simulink model "Sim_Forcing_003h_expe_infra2"  (Simulink 7.4)
settings: Solver=FixedStepDiscrete  StartTime=0.0  StopTime=inf  FixedStep=0.004  RelTol=1e-3
undefined symbols (not defined in the file or in its folder): DiscIntNeverNeededParam
libraries: simulink x42, gt_rt_lib x30, xpcutilitieslib x9, xpclib x2, dspswit3 x1
(part 4 of 5)

== system Sim_Forcing_003h_expe_infra2/Joint Controller (May 7, 2015)/Inverse Kinematics June 22,2016 compatible_minirobot/Simplified Inverse Kinematics/Simplified Inverse Kin ==
  Vec : Inport  OutDataType=fixdt(1, 16)  OutScaling=2^0
  Enable : EnablePort
  Embedded MATLAB Function1 : Stateflow chart
  Out : Outport
  wires:
  Vec/1 -> Embedded MATLAB Function1/1(vec)
  Embedded MATLAB Function1/1(out) -> Out/1

== system Sim_Forcing_003h_expe_infra2/Joint Controller (May 7, 2015)/Inverse Kinematics May 6, 2015/Inverse Kinematics/full inverse kin ==
  vec : Inport
  Enable : EnablePort
  Embedded MATLAB Function : Stateflow chart
  out : Outport  OutDataType=fixdt(1, 16)  OutScaling=2^0
  wires:
  vec/1 -> Embedded MATLAB Function/1(vec)
  Embedded MATLAB Function/1(out) -> out/1

== system Sim_Forcing_003h_expe_infra2/Joint Controller (May 7, 2015)/Inverse Kinematics May 6, 2015/Simplified Inverse Kinematics/A1-A6 COM ==
  vec : Inport
  Demux1 : Demux  Outputs=7
  Ground : Ground
  Ground1 : Ground
  Ground2 : Ground
  Mux1 : Mux  Inputs=6
  Terminator{,1..3} (4 alike) : Terminator
  A1-A6 COM : Outport
  wires:
  Demux1/2 -> Mux1/2
  Demux1/3 -> Mux1/3
  Demux1/5 -> Mux1/5
  Ground/1 -> Mux1/1
  Ground1/1 -> Mux1/4
  Ground2/1 -> Mux1/6
  Demux1/1 -> Terminator/1
  Demux1/4 -> Terminator1/1
  Demux1/6 -> Terminator2/1
  Demux1/7 -> Terminator3/1
  Mux1/1 -> A1-A6 COM/1
  vec/1 -> Demux1/1

== system Sim_Forcing_003h_expe_infra2/Joint Controller (May 7, 2015)/Inverse Kinematics May 6, 2015/Simplified Inverse Kinematics/Simplified Inverse Kin ==
  Vec : Inport  OutDataType=fixdt(1, 16)  OutScaling=2^0
  Enable : EnablePort
  Embedded MATLAB Function1 : Stateflow chart
  Out : Outport
  wires:
  Vec/1 -> Embedded MATLAB Function1/1(vec)
  Embedded MATLAB Function1/1(out) -> Out/1

== matlab function Breaking_Control 20/07/15/Move UP1/add x_offset/Embedded MATLAB Function ==
  data: dx input double; set_out output double; set_in input double
function set_out = add_x_offset(dx, set_in)
%#eml

set_out = set_in;
set_out(3,1) = set_in(3,1) + dx;

== matlab function Breaking_Control 20/07/15/Timeline/Embedded MATLAB Function ==
  data: u input double; y output double; flag_in input double; ac_in input double; ac_out output double
function [y,ac_out]  = fcn(u,flag_in,ac_in)
%#eml
ac_out=ac_in;

if(u>0.2)
    ac_out=1;
    y=1;
else
if(ac_out==1)
    y=1;
    ac_out=1;
else
    y=0;
    ac_out=0;
end    
end

if(flag_in==1)
    ac_out=0;
    y=0;    
end



end

== matlab function Breaking_Control 20/07/15/Embedded MATLAB Function2 ==
  data: com_or input double; T output double size=1; threshold input double; flag_z output double
function [T,flag_z]  = check_angle(com_or,threshold)
%#eml
sum=com_or(1)+com_or(2)+com_or(3);

if(abs(sum)>threshold)
    T=10;
    flag_z=1;
else
    T=5;
    flag_z=0;
    
end

== matlab function Breaking_Control 20/07/15/Timeline/Embedded MATLAB Function2 ==
  data: stim_time input double; t_bool output uint8 size=1; flag_z input double
function t_bool   = adjust_time(stim_time,flag_z)
%#eml

if(flag_z)
    if(stim_time<50)
        t_bool=true;
    else
        t_bool=false;
    end
    
else
    if(stim_time<40)
        t_bool=true;
    else
        t_bool=false;
    end
  
end

== matlab function Joint Controller (May 7, 2015)/Forward Kinematics/Embedded MATLAB Function ==
  data: vec input double; out output uint8
function out = ForKinSim( vec )
%--------------------------------------------------------------------------
%
%   This function solves the FORWARD kinematics of the 6-DOF KUKA arm and
%   wrist. This is the  version,
%   embedded in Simulink. The input and output are vectors that include the
%   list of parameters as defined herafter
%
%       *** Input variables, vec(1:13) ***
%
%   vec(1: 3)    POS         Room coordinates of flange, NED in cm
%   vec(4: 6)    EUL_ANG     Euler angles of the flange, phi, theta, psi, in deg
%   vec(1:6)     J_ANG_0     The joint angles, in deg
%
%       *** Output Variables ***
%
%   out(1: 3)    POS         Room coordinates of flange, NED in cm
%   out(4: 6)    EUL_ANG     Euler angles of the flange, phi, theta, psi, in deg
%
%   The North_East_Down convention is used and psi, theta, phi rotation
%   sequence; A2, A3, A5 are up positive and A4, A6 right rotation positive
%   Note that this is different from the KUKA convention
%
%   Written by Arthur J. Grunwald, Nov. 23, 2014
%
%--------------------------------------------------------------------------
%#eml

DTR = pi/180.;
RTD = 180/pi;

% reload variables
% the algorithm works in rad, so ang is in rad
J_ANG       = vec(1:6);   % Initial guess of the joint angles, in deg
ang         = J_ANG*DTR;

% reserve place for output
out = zeros(6,1);

% define length of arms
l1          = 50.;   % arm length in cm
l2          = 130.;
l3          = 66.;
l4          = 36.5;
l5          = 29.;
d           = 5.5;             % vertical offset of the center line of
% joint 4 from centerline of arm A3
Height_A2   = 104.5 + 106;     % height link A2 above the ground


% 4x4 Transfer matrices, include both rotation and translation

ang = adjust_ang( ang ); % ang is brought in the range +-pi
A1 = ang(1);
A2 = ang(2);
A3 = ang(3);
A4 = ang(4);
A5 = ang(5);
A6 = ang(6);

CA1 = cos(A1);
SA1 = sin(A1);
CA2 = cos(A2);
SA2 = sin(A2);
CA3 = cos(A3);
SA3 = sin(A3);
CA4 = cos(A4);
SA4 = sin(A4);
CA5 = cos(A5);
SA5 = sin(A5);
CA6 = cos(A6);
SA6 = sin(A6);

D1 = [CA1 -SA1 0 0; SA1 CA1 0 0; 0 0 1 0;  0 0 0 1];
D2 = [CA2 0 SA2 l1; 0 1 0 0; -SA2 0 CA2 0; 0 0 0 1];
D3 = [CA3 0 SA3 l2; 0 1 0 0; -SA3 0 CA3 0; 0 0 0 1];
D4 = [1 0 0 l3; 0 CA4 -SA4 0; 0 SA4 CA4 d; 0 0 0 1];
D5 = [CA5 0 SA5 l4; 0 1 0 0; -SA5 0 CA5 0; 0 0 0 1];
D6 = [1 0 0 l5; 0 CA6 -SA6 0; 0 SA6 CA6 0; 0 0 0 1];

% cut out the 3x3 DCM's for each of the transfer matrices
% Note that the DCM is for rotation from b->e
E1 = D1(1:3,1:3);
E2 = D2(1:3,1:3);
E3 = D3(1:3,1:3);
E4 = D4(1:3,1:3);
E5 = D5(1:3,1:3);
E6 = D6(1:3,1:3);

% --- computed position from links A1-A6 ---

x_cabin = [0; 0; 0];    % x,y,z cabin reference point (cm)
% to which the translation is made
x6 = [x_cabin; 1];
p = D1*D2*D3*D4*D5*D6*x6;
pos = p(1:3);        % position of the cabin reference point in the
% NED system (cm)

% computed Euler angles from links A1-A6
% Euler matrices for rotation from e->b (note the transpose)
E = E6'*E5'*E4'*E3'*E2'*E1';
eul_ang = DCM2Eul( E );

% place into output vector
out(1:3,1) = pos-[0;0;Height_A2];
out(4:6,1) = RTD*eul_ang;

end

== matlab function Joint Controller (May 7, 2015)/Inverse Kinematics May 6, 2015/Inverse Kinematics/full inverse kin/Embedded MATLAB Function ==
  data: vec input double; out output double
function out = InvKinSim( vec )
%--------------------------------------------------------------------------
%
%   This function solves the inverse kinematics of the 6-DOF KUKA arm and
%   wrist by means of an iterative algorithm. This is the  version,
%   embedded in Simulink. The input and output are vectors that include the
%   list of parameters as defined herafter
%
%       *** Input variables, vec(1:13) ***
%
%   vec(1: 3)    POS         Room coordinates of flange, NED in cm
%   vec(4: 6)    EUL_ANG     Euler angles of the flange, phi, theta, psi, in deg
%   vec(7:12)    J_ANG_0     Initial guess of the joint angles, in deg
%
%       *** Output Variables ***
%
%   out(1:6)  J_ANG          The six joint angles after convergence
%   out(7)    N, error code  Number of iterations, when negative, it is an
%                            error code:
%                               -1 no convergence
%                               -2 out of reach of joints
%                               -3 joint angles exceeded
%
%   The North_East_Down convention is used and psi, theta, phi rotation
%   sequence; A2, A3, A5 are up positive and A4, A6 right rotation positive
%   Note that this is different from the KUKA convention
%
%   Written by Arthur J. Grunwald, Nov. 14, 2014
%   Re-written for Simulink embedded, Nov. 20, 2014
%
%--------------------------------------------------------------------------
%#eml
DTR = pi/180.;
RTD = 180/pi;

% reload variables
POS         = vec(1: 3);   % Room coordinates of flange, NED in cm
EUL_ANG     = vec(4: 6);   % Euler angles of the flange, phi, theta, psi, in deg
J_ANG_0     = vec(7:12);   % Initial guess of the joint angles, in deg
out         = zeros(7,1);  % reserve place for out

% soft limits on the links (NED convention)

% SL = [   175    130     88    200    61    200
%         -175    -20    -88   -200   -61   -200];

% Dec. 6, 2014: A2 and A3 limits changed to KUKA hardware
% May 7,2015 soft limits on the links (NED convention)
SL = [   159    129     87      349    60    349
        -159    -19    -87     -349   -60   -349];

% define length of arms
l1          = 50.;   % arm length in cm
l2          = 130.;
l3          = 66.;
l4          = 36.5;
l5          = 29.;
d           = 5.5;             % vertical offset of the center line of
% joint 4 from centerline of arm A3
Height_A2   = 104.5 + 106;     % height link A2 above the ground

% offset the height so that level zero is now at the height of the A2 joint
POS(3) = POS(3) + Height_A2;

% set initial guess; the algorithm works in rad, so ang is in rad
N = 0;
ang = J_ANG_0*DTR;

% check for maximum range of arm links and exit with n = 2 when exceeded
L = l2 + l3 + l4 + l5;
R = sqrt(L^2 - POS(3)^2) + l1;
R1 = sqrt(POS(1)^2 + POS(2)^2);
if R1 > R-5;
    out(1:6,1) = J_ANG_0; % return vector as is
    out(7,1)   = -2;
    return
end

%--------------------------------
% 	start of iterative loop
%--------------------------------

while(1)
    
    % 4x4 Transfer matrices, include both rotation and translation
    
    ang = adjust_ang( ang ); % ang is brought in the range +-pi
    A1 = ang(1);
    A2 = ang(2);
    A3 = ang(3);
    A4 = ang(4);
    A5 = ang(5);
    A6 = ang(6);
    
    CA1 = cos(A1);
    SA1 = sin(A1);
    CA2 = cos(A2);
    SA2 = sin(A2);
    CA3 = cos(A3);
    SA3 = sin(A3);
    CA4 = cos(A4);
    SA4 = sin(A4);
    CA5 = cos(A5);
    SA5 = sin(A5);
    CA6 = cos(A6);
    SA6 = sin(A6);
    
    D1 = [CA1 -SA1 0 0; SA1 CA1 0 0; 0 0 1 0;  0 0 0 1];
    D2 = [CA2 0 SA2 l1; 0 1 0 0; -SA2 0 CA2 0; 0 0 0 1];
    D3 = [CA3 0 SA3 l2; 0 1 0 0; -SA3 0 CA3 0; 0 0 0 1];
    D4 = [1 0 0 l3; 0 CA4 -SA4 0; 0 SA4 CA4 d; 0 0 0 1];
    D5 = [CA5 0 SA5 l4; 0 1 0 0; -SA5 0 CA5 0; 0 0 0 1];
    D6 = [1 0 0 l5; 0 CA6 -SA6 0; 0 SA6 CA6 0; 0 0 0 1];
    
    % cut out the 3x3 DCM's for each of the transfer matrices
    % Note that the DCM is for rotation from b->e
    E1 = D1(1:3,1:3);
    E2 = D2(1:3,1:3);
    E3 = D3(1:3,1:3);
    E4 = D4(1:3,1:3);
    E5 = D5(1:3,1:3);
    E6 = D6(1:3,1:3);
    
    % --- computed position from links A1-A6 ---
    
    %----------------------------------------------------------------------
    %   In order to move a point in the cabine in 6-DOF rather than the
    %   endplate, define the coordinates of that point in x_cabin
    %----------------------------------------------------------------------
    x_cabin = [0; 0; 0];    % x,y,z cabin reference point (cm)
    
    x6 = [x_cabin; 1];
    p = D1*D2*D3*D4*D5*D6*x6;
    pos = p(1:3);           % position of the cabin reference point in the
    % NED system (cm)
    
    % computed Euler angles from links A1-A6
    % Euler matrices for rotation from e->b (note the transpose)
    E = E6'*E5'*E4'*E3'*E2'*E1';
    eul_ang = DCM2Eul( E );
    
    % determine the vectors of rotation of the endplate in e-system
    % for each one of the links; this is a 3x6 matrix, when multiplied
    % with the vector of the joint angles, it will give the vector
    % of rotation of the endplate (and also of the cabin reference point)
    % in the NED system
    
    e6 = E1*E2*E3*E4*E5*[1 0 0]'; % x-axis
    e5 = E1*E2*E3*E4*   [0 1 0]'; % y-axis
    e4 = E1*E2*E3*      [1 0 0]'; % x-axis
    e3 = E1*E2*         [0 1 0]'; % y-axis
    e2 = E1*            [0 1 0]'; % y-axis
    e1 = eye(3)*        [0 0 1]'; % z-axis
    
    e = [e1 e2 e3 e4 e5 e6];
    
    % in order to see the changes in phi, theta, psi that this rotation
    % vector causes, we have to transform e->b first in yaw and after that
    % in pitch
    cs_psi = cos(eul_ang(3));
    sn_psi = sin(eul_ang(3));
    cs_tet = cos(eul_ang(2));
    sn_tet = sin(eul_ang(2));
    
    PSI = [cs_psi sn_psi 0; -sn_psi cs_psi 0; 0 0 1];
    TET = [cs_tet 0 -sn_tet; 0 1 0; sn_tet 0 cs_tet];
    e = TET*PSI*e;
    
    
    
    % the derivatives of D1-D6 for eah one of the link angles
    dD1 = [-SA1 -CA1 0 0; CA1 -SA1 0 0; 0 0 0 0; 0 0 0 0];
    dD2 = [-SA2 0 CA2 0; 0 0 0 0; -CA2 0 -SA2 0; 0 0 0 0];
    dD3 = [-SA3 0 CA3 0; 0 0 0 0; -CA3 0 -SA3 0; 0 0 0 0];
    dD4 = [0 0 0 0; 0 -SA4 -CA4 0; 0 CA4 -SA4 0; 0 0 0 0];
    dD5 = [-SA5 0 CA5 0; 0 0 0 0; -CA5 0 -SA5 0; 0 0 0 0];
    dD6 = [0 0 0 0; 0 -SA6 -CA6 0; 0 CA6 -SA6 0; 0 0 0 0];
    
    % Hessian Matrix H; the inverse of this matrix determines the link
    % angle speed as a function of the speed of x,y,z and the speed of the
    % Euler angles
    
    h1 = dD1*D2*D3*D4*D5*D6*x6;
    h2 = D1*dD2*D3*D4*D5*D6*x6;
    h3 = D1*D2*dD3*D4*D5*D6*x6;
    h4 = D1*D2*D3*dD4*D5*D6*x6;
    h5 = D1*D2*D3*D4*dD5*D6*x6;
    h6 = D1*D2*D3*D4*D5*dD6*x6;
    
    h = [h1 h2 h3 h4 h5 h6]; % this 3x6 is th upper half of H
    H = [h(1:3,:); e];       % the lower 3x6 half is the matrix e
    
    d_ang = inv(H) * [( POS - pos ); (DTR*EUL_ANG - eul_ang)];
    ang = ang + d_ang;
    ang = adjust_ang( ang );
    if(norm(d_ang) < 1.e-6)
        J_ANG = RTD*adjust_ang( ang );
        out(1:6,1) = J_ANG;
        out(7,1)   = N;
        break;
    end
    N = N + 1;
    
    % if more than 10 iterations, no convergence
    if N > 10
        out(1:6) = J_ANG_0; % return vector as is
        out(7)   = -1;
        return;
    end
end

% tests whether the links are within the set soft limits
for i = 1 : 6
    if J_ANG(i) >= SL(1,i)
        out(7,1) = -3;
        return;
    elseif J_ANG(i) <= SL(2,i)
        out(7,1) = -3;
        return;
    end
end

end

== matlab function Joint Controller (May 7, 2015)/Inverse Kinematics May 6, 2015/Simplified Inverse Kinematics/Simplified Inverse Kin/Embedded MATLAB Function1 ==
  data: vec input double; out output double
function out = SimpleInvKin( vec )

% We use the NED convention
% This algorithm has a closed form solution and is based on the cosine rule
% However, due to the offset of the centerline of link A4 55 mm below the
% center of rotation of link A3, some small corrections have to be made;
% this is done iteratively by means of a second-order scheme.
% The gist of this routine is to show tha identical results are obtained
% with the fully-fledged 6-DOF inverse algorithm.
%
% The algorithm is also used for computing an initial guess for the
% fully-fledged inverse kinematics algorithm
% The initial guess uses only links A1, A2, A3 and assumes that the
% cabin at the end is straight and level and aligned with the arm
% Thus A4 and A6 are zero and A5 is A2 + A3
%
%   out(7) includes the parameter N
%       N > 0           the number of iterations needed to converge
%       N = -1          the iterative algorithm does not converge
%       N = -2          out of reachable limits
%       N -10<N<-30     upper limit of one of the joints A1-A6 exceeded
%       N -100<N<-110   upper limit of one of the joints A1-A6 exceeded
%
%   Written by Arthur Grunwald, November 11, 2014
%   Added correction because of offset of link A4, Dec 2, 2014
%   Added theta degree-of-freedom April 14, 2015
%   Modified the iterative scheme to second order NR scheme April 24, 2015
%   Modified FAR and CLOSE checks with intersecting circles May 6, 2015

RTD = 180/pi;
DTR = pi/180;

% May 7,2015 soft limits on the links (NED convention)
SL = [   159    129     87      349    60    349
        -159    -19    -87     -349   -60   -349];

% define length of the links

l1          = 50.;   % arm length in cm
l2          = 130.;
l3          = 66.;
l4          = 36.5;
l5          = 29.;
offset      = 5.5;             % vertical offset of the center line of
% joint 4 from centerline of arm A3
% joint 4 from centerline of arm A3
Height_A2   = 104.5 + 106;     % height link A2 above the ground

x = vec(1);
y = vec(2);
z = vec(3);

theta = vec(5);
cos_theta = cos(DTR*vec(5));
sin_theta = sin(DTR*vec(5));

N = 1;
out = zeros(7,1);

% compute dimensions of triangle
l = sqrt(x*x + y*y);
e = l - l1 - l5*cos_theta;
h = -(Height_A2 + z)-l5*sin_theta;
d = sqrt(e^2 + h^2);

% check whether the FAR location of C is reachable
b = l2;
c = l3 + l4;
margin = 5; % margin is 5 cm
if d > b + c - margin
    out(1:6,1) = vec(7:12); % return angles 'as is'
    out(3,1) = -90;
    out(7,1) = -2;
    return
end

% check whether the CLOSE location of C is reachable
if d + c - margin < b
    out(1:6,1) = vec(7:12); % return angles 'as is'
    out(3,1) = -90;
    out(7,1) = -2;
    return
end

% This iterative loop serves to correct for the offset of link A4
% A first good guess is to assume that beta is initially 90 deg
% A second-order scheme is used

A3 = vec(9);
beta = A3 + 180.;

while(1)
    
    sin_beta = sin(beta*DTR);
    sin2_beta = sin_beta*sin_beta;
    cos_beta = cos(beta*DTR);
    
    b = l2 - offset/sin_beta;
    c = l3 + l4 - offset*cos_beta/sin_beta;
    
    db_dbeta = offset * cos_beta/sin2_beta;
    dc_dbeta = offset/sin2_beta;
    
    A = (b*b + c*c - d*d);
    B = (2*b*c);
    dA_dbeta = (2*b*db_dbeta + 2*c*dc_dbeta);
    dB_dbeta = 2*(db_dbeta*c + b*dc_dbeta);
    eps = cos_beta - A/B;
    deps_dbeta = -sin_beta - (dA_dbeta*B - A*dB_dbeta)/B^2;
    dbeta = -RTD*eps/deps_dbeta;
    beta = beta + dbeta;
    
    if abs(dbeta) < 1.e-5
        break
    end
    N = N + 1;
    if N > 100
        N = -2;
        out(1:6,1) = vec(7:12); % return angles 'as is'
        out(3,1) = -90;
        out(7,1) = N;
        break;
    end
end

% employ cosine rule on angles alpha and beta of triangle
cos_alpha = (b*b + d*d - c*c)/(2*b*d);

alpha = RTD*acos(cos_alpha);
delta = RTD*atan2(h, e);

% the link angles
A1 = RTD*atan2(y, x);
A2 = alpha + delta;
A3 = beta - 180;
A4 = 0;
A5 = -(A2 + A3) + theta;
A6 = 0;

J_ANG = [A1 A2 A3 A4 A5 A6]';
out(1:6,1) = J_ANG;

% tests whether the links are within the set soft limits
for i = 1 : 6
    if J_ANG(i) >= SL(1,i)
        N = -10-i;
    elseif J_ANG(i) <= SL(2,i)
        N = -100-i;
    end
end

out(7,1) = N;

end

== matlab function Breaking_Control 20/07/15/Move UP1/curve ==
  data: set input double; psi_set input double; x output double; fraction input double; z output double; psi output double; c output double; z_p output double
function [x, z, psi, c, z_p] = curve(set, psi_set, fraction)
%#eml
%**************************************************************************
%
% for fitting a parabolic curve through 3 points
%
%   set is a 3 x 2 matrix that include:
%       (x1, z1)
%       (x2, z2)
%       (x3, z3)
%
%   z is the abcis and x the ordinate of the curve
%   fraction runs from 0 to 1
%
%**************************************************************************

z_p = set(:,2);
x_p = set(:,1);

A = [z_p.*z_p z_p ones(3,1)];
c = A\x_p;

z = fraction*(z_p(3) - z_p(1)) + z_p(1);

x = [z.*z z 1]*c;

psi = fraction * psi_set;

== matlab function Joint Controller (May 7, 2015)/Inverse Kinematics June 22,2016 compatible_minirobot/Embedded MATLAB Function ==
  data: J_ANG_COURANTS input double; SCALED_J_ANG output double; J_ANG_ANCIENS input double
function SCALED_J_ANG  = LimitesCinematiqes(J_ANG_COURANTS, J_ANG_ANCIENS)
%#eml

A1C=J_ANG_COURANTS(1);      A1A=J_ANG_ANCIENS(1);
A2C=J_ANG_COURANTS(2);      A2A=J_ANG_ANCIENS(2);
A3C=J_ANG_COURANTS(3);      A3A=J_ANG_ANCIENS(3);
A4C=J_ANG_COURANTS(4);      A4A=J_ANG_ANCIENS(4);
A5C=J_ANG_COURANTS(5);      A5A=J_ANG_ANCIENS(5);
A6C=J_ANG_COURANTS(6);      A6A=J_ANG_ANCIENS(6);

BCtheta1=0.2734; BCtheta2=0.228; BCtheta3=0.276;
BCtheta45=0.304; BCtheta6=0.48;   
%---THETA1----------------------
delta1=A1C-A1A;
if(abs(delta1)> BCtheta1)
    Theta1=A1A+sign(delta1)*BCtheta1;
else
    Theta1=A1C;
end

%---THETA2----------------------
delta2=A2C-A2A;
if(abs(delta2)> BCtheta2)
    Theta2=A2A+sign(delta2)*BCtheta2;
else
    Theta2=A2C;
end
%---THETA3----------------------
delta3=A3C-A3A;
if(abs(delta3)> BCtheta3)
    Theta3=A3A+sign(delta3)*BCtheta3;
else
    Theta3=A3C;
end

%---THETA4----------------------
delta4=A4C-A4A;
if(abs(delta4)> BCtheta45)
    Theta4=A4A+sign(delta4)*BCtheta45;
else
    Theta4=A4C;
end
%---THETA5----------------------
delta5=A5C-A5A;
if(abs(delta5)> BCtheta45)
    Theta5=A5A+sign(delta5)*BCtheta45;
else
    Theta5=A5C;
end
%---THETA6----------------------
delta6=A6C-A6A;
if(abs(delta6)> BCtheta6)
    Theta6=A6A+sign(delta6)*BCtheta6;
else
    Theta6=A6C;
end
SCALED_J_ANG=[Theta1, Theta2, Theta3, Theta4, Theta5, Theta6];
end

== matlab function Breaking_Control 20/07/15/Timeline/Embedded MATLAB Function1 ==
  data: stim_time input double; t_bool output double size=1; flag_z input double
function t_bool   = adjust_time(stim_time,flag_z)
%#eml

if(flag_z)
    if(stim_time>=50)
        t_bool=true;
    else
        t_bool=false;
    end
    
else
    if(stim_time>=40)
        t_bool=true;
    else
        t_bool=false;
    end
  
end

== matlab function Breaking_Control 20/07/15/Timeline/Embedded MATLAB Function3 ==
  data: stim_time input double; t_bool output double size=1; flag_z input double
function t_bool   = adjust_time(stim_time,flag_z)
%#eml

if(flag_z)
    if(stim_time>=60)
        t_bool=true;
    else
        t_bool=false;
    end
    
else
    if(stim_time>=50)
        t_bool=true;
    else
        t_bool=false;
    end
  
end

== matlab function Breaking_Control 20/07/15/Timeline/Embedded MATLAB Function4 ==
  data: stim_time input double; t_bool output double size=1; flag_z input double
function t_bool   = adjust_time(stim_time,flag_z)
%#eml

if(flag_z)
    if(stim_time<30)
        t_bool=true;
    else
        t_bool=false;
    end
    
else
    if(stim_time<20)
        t_bool=true;
    else
        t_bool=false;
    end
  
end

== matlab function Joint Controller (May 7, 2015)/Inverse Kinematics June 22,2016 compatible_minirobot/Inverse Kinematics/full inverse kin/Embedded MATLAB Function ==
  data: vec input double; out output double
function out = InvKinSim( vec )
%--------------------------------------------------------------------------
%
%   This function solves the inverse kinematics of the 6-DOF KUKA arm and
%   wrist by means of an iterative algorithm. This is the  version,
%   embedded in Simulink. The input and output are vectors that include the
%   list of parameters as defined herafter
%
%       *** Input variables, vec(1:13) ***
%
%   vec(1: 3)    POS         Room coordinates of flange, NED in cm
%   vec(4: 6)    EUL_ANG     Euler angles of the flange, phi, theta, psi, in deg
%   vec(7:12)    J_ANG_0     Initial guess of the joint angles, in deg
%
%       *** Output Variables ***
%
%   out(1:6)  J_ANG          The six joint angles after convergence
%   out(7)    N, error code  Number of iterations, when negative, it is an
%                            error code:
%                               -1 no convergence
%                               -2 out of reach of joints
%                               -3 joint angles exceeded
%
%   The North_East_Down convention is used and psi, theta, phi rotation
%   sequence; A2, A3, A5 are up positive and A4, A6 right rotation positive
%   Note that this is different from the KUKA convention
%
%   Written by Arthur J. Grunwald, Nov. 14, 2014
%   Re-written for Simulink embedded, Nov. 20, 2014
%
%--------------------------------------------------------------------------
%#eml
DTR = pi/180.;
RTD = 180/pi;

% reload variables
POS         = vec(1: 3);   % Room coordinates of flange, NED in cm
EUL_ANG     = vec(4: 6);   % Euler angles of the flange, phi, theta, psi, in deg
J_ANG_0     = vec(7:12);   % Initial guess of the joint angles, in deg
out         = zeros(7,1);  % reserve place for out

% soft limits on the links (NED convention)

% SL = [   175    130     88    200    61    200
%         -175    -20    -88   -200   -61   -200];

% Dec. 6, 2014: A2 and A3 limits changed to KUKA hardware
% May 7,2015 soft limits on the links (NED convention)
SL = [   159    129     87      349    60    349
        -159    -19    -87     -349   -60   -349];

% define length of arms
l1          = 50.;   % arm length in cm
l2          = 130.;
l3          = 66.;
l4          = 36.5;
l5          = 29.;
d           = 5.5;             % vertical offset of the center line of
% joint 4 from centerline of arm A3
Height_A2   = 104.5 + 106;     % height link A2 above the ground

% offset the height so that level zero is now at the height of the A2 joint
POS(3) = POS(3) + Height_A2;

% set initial guess; the algorithm works in rad, so ang is in rad
N = 0;
ang = J_ANG_0*DTR;

% check for maximum range of arm links and exit with n = 2 when exceeded
L = l2 + l3 + l4 + l5;
R = sqrt(L^2 - POS(3)^2) + l1;
R1 = sqrt(POS(1)^2 + POS(2)^2);
if R1 > R-5;
    out(1:6,1) = J_ANG_0; % return vector as is
    out(7,1)   = -2;
    return
end

%--------------------------------
% 	start of iterative loop
%--------------------------------

while(1)
    
    % 4x4 Transfer matrices, include both rotation and translation
    
    ang = adjust_ang( ang ); % ang is brought in the range +-pi
    A1 = ang(1);
    A2 = ang(2);
    A3 = ang(3);
    A4 = ang(4);
    A5 = ang(5);
    A6 = ang(6);
    
    CA1 = cos(A1);
    SA1 = sin(A1);
    CA2 = cos(A2);
    SA2 = sin(A2);
    CA3 = cos(A3);
    SA3 = sin(A3);
    CA4 = cos(A4);
    SA4 = sin(A4);
    CA5 = cos(A5);
    SA5 = sin(A5);
    CA6 = cos(A6);
    SA6 = sin(A6);
    
    D1 = [CA1 -SA1 0 0; SA1 CA1 0 0; 0 0 1 0;  0 0 0 1];
    D2 = [CA2 0 SA2 l1; 0 1 0 0; -SA2 0 CA2 0; 0 0 0 1];
    D3 = [CA3 0 SA3 l2; 0 1 0 0; -SA3 0 CA3 0; 0 0 0 1];
    D4 = [1 0 0 l3; 0 CA4 -SA4 0; 0 SA4 CA4 d; 0 0 0 1];
    D5 = [CA5 0 SA5 l4; 0 1 0 0; -SA5 0 CA5 0; 0 0 0 1];
    D6 = [1 0 0 l5; 0 CA6 -SA6 0; 0 SA6 CA6 0; 0 0 0 1];
    
    % cut out the 3x3 DCM's for each of the transfer matrices
    % Note that the DCM is for rotation from b->e
    E1 = D1(1:3,1:3);
    E2 = D2(1:3,1:3);
    E3 = D3(1:3,1:3);
    E4 = D4(1:3,1:3);
    E5 = D5(1:3,1:3);
    E6 = D6(1:3,1:3);
    
    % --- computed position from links A1-A6 ---
    
    %----------------------------------------------------------------------
    %   In order to move a point in the cabine in 6-DOF rather than the
    %   endplate, define the coordinates of that point in x_cabin
    %----------------------------------------------------------------------
    x_cabin = [0; 0; 0];    % x,y,z cabin reference point (cm)
    
    x6 = [x_cabin; 1];
    p = D1*D2*D3*D4*D5*D6*x6;
    pos = p(1:3);           % position of the cabin reference point in the
    % NED system (cm)
    
    % computed Euler angles from links A1-A6
    % Euler matrices for rotation from e->b (note the transpose)
    E = E6'*E5'*E4'*E3'*E2'*E1';
    eul_ang = DCM2Eul( E );
    
    % determine the vectors of rotation of the endplate in e-system
    % for each one of the links; this is a 3x6 matrix, when multiplied
    % with the vector of the joint angles, it will give the vector
    % of rotation of the endplate (and also of the cabin reference point)
    % in the NED system
    
    e6 = E1*E2*E3*E4*E5*[1 0 0]'; % x-axis
    e5 = E1*E2*E3*E4*   [0 1 0]'; % y-axis
    e4 = E1*E2*E3*      [1 0 0]'; % x-axis
    e3 = E1*E2*         [0 1 0]'; % y-axis
    e2 = E1*            [0 1 0]'; % y-axis
    e1 = eye(3)*        [0 0 1]'; % z-axis
    
    e = [e1 e2 e3 e4 e5 e6];
    
    % in order to see the changes in phi, theta, psi that this rotation
    % vector causes, we have to transform e->b first in yaw and after that
    % in pitch
    cs_psi = cos(eul_ang(3));
    sn_psi = sin(eul_ang(3));
    cs_tet = cos(eul_ang(2));
    sn_tet = sin(eul_ang(2));
    
    PSI = [cs_psi sn_psi 0; -sn_psi cs_psi 0; 0 0 1];
    TET = [cs_tet 0 -sn_tet; 0 1 0; sn_tet 0 cs_tet];
    e = TET*PSI*e;
    
    
    
    % the derivatives of D1-D6 for eah one of the link angles
    dD1 = [-SA1 -CA1 0 0; CA1 -SA1 0 0; 0 0 0 0; 0 0 0 0];
    dD2 = [-SA2 0 CA2 0; 0 0 0 0; -CA2 0 -SA2 0; 0 0 0 0];
    dD3 = [-SA3 0 CA3 0; 0 0 0 0; -CA3 0 -SA3 0; 0 0 0 0];
    dD4 = [0 0 0 0; 0 -SA4 -CA4 0; 0 CA4 -SA4 0; 0 0 0 0];
    dD5 = [-SA5 0 CA5 0; 0 0 0 0; -CA5 0 -SA5 0; 0 0 0 0];
    dD6 = [0 0 0 0; 0 -SA6 -CA6 0; 0 CA6 -SA6 0; 0 0 0 0];
    
    % Hessian Matrix H; the inverse of this matrix determines the link
    % angle speed as a function of the speed of x,y,z and the speed of the
    % Euler angles
    
    h1 = dD1*D2*D3*D4*D5*D6*x6;
    h2 = D1*dD2*D3*D4*D5*D6*x6;
    h3 = D1*D2*dD3*D4*D5*D6*x6;
    h4 = D1*D2*D3*dD4*D5*D6*x6;
    h5 = D1*D2*D3*D4*dD5*D6*x6;
    h6 = D1*D2*D3*D4*D5*dD6*x6;
    
    h = [h1 h2 h3 h4 h5 h6]; % this 3x6 is th upper half of H
    H = [h(1:3,:); e];       % the lower 3x6 half is the matrix e
    
    d_ang = inv(H) * [( POS - pos ); (DTR*EUL_ANG - eul_ang)];
    ang = ang + d_ang;
    ang = adjust_ang( ang );
    if(norm(d_ang) < 1.e-6)
        J_ANG = RTD*adjust_ang( ang );
        out(1:6,1) = J_ANG;
        out(7,1)   = N;
        break;
    end
    N = N + 1;
    
    % if more than 10 iterations, no convergence
    if N > 10
        out(1:6) = J_ANG_0; % return vector as is
        out(7)   = -1;
        return;
    end
end

% tests whether the links are within the set soft limits
for i = 1 : 6
    if J_ANG(i) >= SL(1,i)
        out(7,1) = -3;
        return;
    elseif J_ANG(i) <= SL(2,i)
        out(7,1) = -3;
        return;
    end
end

end

== matlab function Joint Controller (May 7, 2015)/Inverse Kinematics June 22,2016 compatible_minirobot/Inverse Kinematics mini robot/full inverse kin/Embedded MATLAB Function ==
  data: vec input double; out output double
function out = InvKinSim( vec )
%--------------------------------------------------------------------------
%
%   This function solves the inverse kinematics of the 6-DOF KUKA arm and
%   wrist by means of an iterative algorithm. This is the  version,
%   embedded in Simulink. The input and output are vectors that include the
%   list of parameters as defined herafter
%
%       *** Input variables, vec(1:13) ***
%
%   vec(1: 3)    POS         Room coordinates of flange, NED in cm
%   vec(4: 6)    EUL_ANG     Euler angles of the flange, phi, theta, psi, in deg
%   vec(7:12)    J_ANG_0     Initial guess of the joint angles, in deg
%
%       *** Output Variables ***
%
%   out(1:6)  J_ANG          The six joint angles after convergence
%   out(7)    N, error code  Number of iterations, when negative, it is an
%                            error code:
%                               -1 no convergence
%                               -2 out of reach of joints
%                               -3 joint angles exceeded
%
%   The North_East_Down convention is used and psi, theta, phi rotation
%   sequence; A2, A3, A5 are up positive and A4, A6 right rotation positive
%   Note that this is different from the KUKA convention
%
%   Written by Arthur J. Grunwald, Nov. 14, 2014
%   Re-written for Simulink embedded, Nov. 20, 2014
%
%--------------------------------------------------------------------------
%#eml
DTR = pi/180.;
RTD = 180/pi;

% reload variables
POS         = vec(1: 3);   % Room coordinates of flange, NED in cm
EUL_ANG     = vec(4: 6);   % Euler angles of the flange, phi, theta, psi, in deg
J_ANG_0     = vec(7:12);   % Initial guess of the joint angles, in deg
out         = zeros(7,1);  % reserve place for out

% soft limits on the links (NED convention)

% SL = [   175    130     88    200    61    200
%         -175    -20    -88   -200   -61   -200];

% Dec. 6, 2014: A2 and A3 limits changed to KUKA hardware
% May 7,2015 soft limits on the links (NED convention)
SL = [   159    129     87      349    60    349
        -159    -19    -87     -349   -60   -349];

% define length of arms
l1          = 50.;   % arm length in cm
l2          = 130.;
l3          = 66.;
l4          = 36.5;
l5          = 29.;
d           = 5.5;             % vertical offset of the center line of
% joint 4 from centerline of arm A3
Height_A2   = 104.5 + 106;     % height link A2 above the ground

% offset the height so that level zero is now at the height of the A2 joint
POS(3) = POS(3) + Height_A2;

% set initial guess; the algorithm works in rad, so ang is in rad
N = 0;
ang = J_ANG_0*DTR;

% check for maximum range of arm links and exit with n = 2 when exceeded
L = l2 + l3 + l4 + l5;
R = sqrt(L^2 - POS(3)^2) + l1;
R1 = sqrt(POS(1)^2 + POS(2)^2);
if R1 > R-5;
    out(1:6,1) = J_ANG_0; % return vector as is
    out(7,1)   = -2;
    return
end

%--------------------------------
% 	start of iterative loop
%--------------------------------

while(1)
    
    % 4x4 Transfer matrices, include both rotation and translation
    
    ang = adjust_ang( ang ); % ang is brought in the range +-pi
    A1 = ang(1);
    A2 = ang(2);
    A3 = ang(3);
    A4 = ang(4);
    A5 = ang(5);
    A6 = ang(6);
    
    CA1 = cos(A1);
    SA1 = sin(A1);
    CA2 = cos(A2);
    SA2 = sin(A2);
    CA3 = cos(A3);
    SA3 = sin(A3);
    CA4 = cos(A4);
    SA4 = sin(A4);
    CA5 = cos(A5);
    SA5 = sin(A5);
    CA6 = cos(A6);
    SA6 = sin(A6);
    
    D1 = [CA1 -SA1 0 0; SA1 CA1 0 0; 0 0 1 0;  0 0 0 1];
    D2 = [CA2 0 SA2 l1; 0 1 0 0; -SA2 0 CA2 0; 0 0 0 1];
    D3 = [CA3 0 SA3 l2; 0 1 0 0; -SA3 0 CA3 0; 0 0 0 1];
    D4 = [1 0 0 l3; 0 CA4 -SA4 0; 0 SA4 CA4 d; 0 0 0 1];
    D5 = [CA5 0 SA5 l4; 0 1 0 0; -SA5 0 CA5 0; 0 0 0 1];
    D6 = [1 0 0 l5; 0 CA6 -SA6 0; 0 SA6 CA6 0; 0 0 0 1];
    
    % cut out the 3x3 DCM's for each of the transfer matrices
    % Note that the DCM is for rotation from b->e
    E1 = D1(1:3,1:3);
    E2 = D2(1:3,1:3);
    E3 = D3(1:3,1:3);
    E4 = D4(1:3,1:3);
    E5 = D5(1:3,1:3);
    E6 = D6(1:3,1:3);
    
    % --- computed position from links A1-A6 ---
    
    %----------------------------------------------------------------------
    %   In order to move a point in the cabine in 6-DOF rather than the
    %   endplate, define the coordinates of that point in x_cabin
    %----------------------------------------------------------------------
    x_cabin = [0; 0; 0];    % x,y,z cabin reference point (cm)
    
    x6 = [x_cabin; 1];
    p = D1*D2*D3*D4*D5*D6*x6;
    pos = p(1:3);           % position of the cabin reference point in the
    % NED system (cm)
    
    % computed Euler angles from links A1-A6
    % Euler matrices for rotation from e->b (note the transpose)
    E = E6'*E5'*E4'*E3'*E2'*E1';
    eul_ang = DCM2Eul( E );
    
    % determine the vectors of rotation of the endplate in e-system
    % for each one of the links; this is a 3x6 matrix, when multiplied
    % with the vector of the joint angles, it will give the vector
    % of rotation of the endplate (and also of the cabin reference point)
    % in the NED system
    
    e6 = E1*E2*E3*E4*E5*[1 0 0]'; % x-axis
    e5 = E1*E2*E3*E4*   [0 1 0]'; % y-axis
    e4 = E1*E2*E3*      [1 0 0]'; % x-axis
    e3 = E1*E2*         [0 1 0]'; % y-axis
    e2 = E1*            [0 1 0]'; % y-axis
    e1 = eye(3)*        [0 0 1]'; % z-axis
    
    e = [e1 e2 e3 e4 e5 e6];
    
    % in order to see the changes in phi, theta, psi that this rotation
    % vector causes, we have to transform e->b first in yaw and after that
    % in pitch
    cs_psi = cos(eul_ang(3));
    sn_psi = sin(eul_ang(3));
    cs_tet = cos(eul_ang(2));
    sn_tet = sin(eul_ang(2));
    
    PSI = [cs_psi sn_psi 0; -sn_psi cs_psi 0; 0 0 1];
    TET = [cs_tet 0 -sn_tet; 0 1 0; sn_tet 0 cs_tet];
    e = TET*PSI*e;
    
    
    
    % the derivatives of D1-D6 for eah one of the link angles
    dD1 = [-SA1 -CA1 0 0; CA1 -SA1 0 0; 0 0 0 0; 0 0 0 0];
    dD2 = [-SA2 0 CA2 0; 0 0 0 0; -CA2 0 -SA2 0; 0 0 0 0];
    dD3 = [-SA3 0 CA3 0; 0 0 0 0; -CA3 0 -SA3 0; 0 0 0 0];
    dD4 = [0 0 0 0; 0 -SA4 -CA4 0; 0 CA4 -SA4 0; 0 0 0 0];
    dD5 = [-SA5 0 CA5 0; 0 0 0 0; -CA5 0 -SA5 0; 0 0 0 0];
    dD6 = [0 0 0 0; 0 -SA6 -CA6 0; 0 CA6 -SA6 0; 0 0 0 0];
    
    % Hessian Matrix H; the inverse of this matrix determines the link
    % angle speed as a function of the speed of x,y,z and the speed of the
    % Euler angles
    
    h1 = dD1*D2*D3*D4*D5*D6*x6;
    h2 = D1*dD2*D3*D4*D5*D6*x6;
    h3 = D1*D2*dD3*D4*D5*D6*x6;
    h4 = D1*D2*D3*dD4*D5*D6*x6;
    h5 = D1*D2*D3*D4*dD5*D6*x6;
    h6 = D1*D2*D3*D4*D5*dD6*x6;
    
    h = [h1 h2 h3 h4 h5 h6]; % this 3x6 is th upper half of H
    H = [h(1:3,:); e];       % the lower 3x6 half is the matrix e
    
    d_ang = inv(H) * [( POS - pos ); (DTR*EUL_ANG - eul_ang)];
    ang = ang + d_ang;
    ang = adjust_ang( ang );
    if(norm(d_ang) < 1.e-6)
        J_ANG = RTD*adjust_ang( ang );
        out(1:6,1) = J_ANG;
        out(7,1)   = N;
        break;
    end
    N = N + 1;
    
    % if more than 10 iterations, no convergence
    if N > 10
        out(1:6) = J_ANG_0; % return vector as is
        out(7)   = -1;
        return;
    end
end

% tests whether the links are within the set soft limits
for i = 1 : 6
    if J_ANG(i) >= SL(1,i)
        out(7,1) = -3;
        return;
    elseif J_ANG(i) <= SL(2,i)
        out(7,1) = -3;
        return;
    end
end

end

== matlab function Joint Controller (May 7, 2015)/Inverse Kinematics June 22,2016 compatible_minirobot/Inverse Kinematics mini robot/full inverse kin/Embedded MATLAB Function1 ==
  data: Input input double; Output output double
function Output = MGI_iteratif( Input )
%#eml
%% Quelques raccourcis:
DTR = pi/180.;  % [°] vers [Rad]
RTD = 180/pi;   % [Rad] vers [°]

%% Initialisation des variables INPUT/OUTPUT:
POS         = Input(1: 3)/7;   % Coordonnées de l'effecteur[cm] Convention NED 
                             % ordre: x, y, z
POS(1)      = POS(1)-4;
POS(2)      = -POS(2);     % Pour passer de NED a KUKA
POS(3)      = -POS(3);     % Pour passer de NED a KUKA

EUL_ANG     = Input(4: 6);   % Angles d'Euler de l'effecteur[°] ordre: phi, theta, psi
J_ANG_0     = Input(7:12);   % Valeurs initiales des angles[°]
Output      = zeros(7,1);    % Allocation mémoire de la sortie

%% Les butées angulaires des articulations (Maquette IMOSE):
SL = [    155   21         145    105   120    100
          - 155    -190    -137    -105     -98     -110 ]; % butées maximales
      % butées minimales    
          

%% Les dimensions des bras du robot (Maquette IMOSE):
% Les valeurs ci-dessous sont exprimées en [cm]
l1    = 0;          % Décalage en x du bras1 par rapport au socle
l2    = 20;         % Distance en le moteur2 et le moteur3
l3    = 16;         % Distance en le moteur3 et le moteur4
l4    = 6;          % Distance en le moteur4 et le moteur5
l5    = 3;          % Distance en le moteur5 et le moteur6
d     = 0.2;        % Décalage entre les axces des moteurs 3 et 4

%% Les offsets nécessaires pour décaler les repères:
Height_A2   = 9.8;    % Offset de décalage du repère monde pour 
                      % la hauteur du socle
                                
POS(3) = POS(3) + Height_A2;    % Offset pour redéfinir le point en fonction 
                                % de la nouvelle position du repère monde

%% Initialisation des variables de l'algorithme
N = 0;              % N définit le nombre de boucles réalisées par l'algorithme
                    % pour trouver une solution
                    
% L'algorithme fonctionne en [Rad]                    
ang = J_ANG_0*DTR;  % ang est un vecteur [6x1] pour les valeurs angulaires
                    % de chaque articulation

%% Mise en place de sécurité: Le point défini est hors de portée du robot
L = l2 + l3 + l4 + l5;              % Longueur maximale du bras total en déplacement
R = sqrt(L^2 - POS(3)^2) + l1;      % 
Norme = sqrt(POS(1)^2 + POS(2)^2);     % Calcul de la norme : racine(x²+z²)

if Norme > R-5;
    Output(1:6,1) = J_ANG_0;   
    Output(7,1)   = -2;             % Code d'erreur: -2 <=> Hors de portée
    return
end
%--------------------------------
% DEBUT DE L'ALGORITHME ITERATIF
%--------------------------------
while(1)
        
    ang = adjust_ang( ang );        % Appel de la fonction "adjust_ang" pour
                                    % que l'angle soit compris dans [-pi,pi]
    
    % Quelques raccourcis pour accéler la vitesse de calcul
    A1 = ang(1);    A2 = ang(2);    A3 = ang(3);
    A4 = ang(4);    A5 = ang(5);    A6 = ang(6);
    
    CA1 = cos(A1);   SA1 = sin(A1);    CA2 = cos(A2);
    SA2 = sin(A2);   CA3 = cos(A3);    SA3 = sin(A3);
    CA4 = cos(A4);   SA4 = sin(A4);    CA5 = cos(A5);
    SA5 = sin(A5);   CA6 = cos(A6);    SA6 = sin(A6);
    
    % Les matrices de tranformations homogènes selon la convention NED
    D1 = [CA1 -SA1  0  0; 
          SA1  CA1  0  0;     % Matrice de passage du repère 0
            0    0  1  0;     % au repère 1
            0    0  0  1];
    
    D2 = [CA2  0 SA2  l1;
            0  1   0   0;     % Matrice de passage du repère 1
         -SA2  0 CA2   0;     % au repère 2
            0  0   0   1];
    
    D3 = [CA3  0 SA3  l2;
            0  1   0   0;     % Matrice de passage du repère 2
         -SA3  0 CA3   0;     % au repère 3
            0  0   0   1];
        
    D4 = [1   0    0  l3;
          0 CA4 -SA4   0;     % Matrice de passage du repère 3
          0 SA4  CA4   0;     % au repère 4
          0   0    0   1];
    
    D5 = [CA5  0  SA5  l4;
            0  1    0   0;    % Matrice de passage du repère 4
         -SA5  0  CA5   d;    % au repère 5
            0  0    0   1];
    
    D6 = [1   0    0  l5; 
          0 CA6 -SA6   0;     % Matrice de passage du repère 5
          0 SA6  CA6   0;     % au repère 6 (organe terminal <=> deffecteur)
          0   0    0   1];
    
    % On conserve uniquement la partie [3x3] (orientation) des matrices de
    % transformations homogènes D1 à D6
    E1 = D1(1:3,1:3);    % Partie orientation de D1
    E2 = D2(1:3,1:3);    % Partie orientation de D2
    E3 = D3(1:3,1:3);    % Partie orientation de D3
    E4 = D4(1:3,1:3);    % Partie orientation de D4
    E5 = D5(1:3,1:3);    % Partie orientation de D5
    E6 = D6(1:3,1:3);    % Partie orientation de D6
    
    % Pour déplacer un point de la cabine selon 6 DDL plutôt que de
    % déplacer l'assiette, définissons les coordonnées du point telles que:
    x_cabin = [0;   % x    Triplet de coordonneés 
               0;   % y    du point de référence 
               0];  % z    de la cabine en [cm]
    
    x6 = [x_cabin;   % Vecteur intermédiaire pour la position
          1];        % de référence du defecteur
      
    p = D1*D2*D3*D4*D5*D6*x6;  % Vecteur intermédiaire pour la position de référence
    pos = p(1:3);              % Position de référence du deffecteur convention NED [cm]
    
    
    % Les angles d'Euler calculés depuis les articulations 1 à 6
    % Les matrices d'Euler pour les rotations futures , noter qu'on les transpose
    E = E6'*E5'*E4'*E3'*E2'*E1';
    
    eul_ang = DCM2Eul( E );   % Appel de la fonction "DCM2Eul" Traduction des 
                              % matrices de cosinus directeurs en angles d'Euler
    
                              
    % Déterminons les cecteurs de rotations e l'assiette dans le système "e" 
    % pour chacune de articulations. Il s'agit d'une matrice [3x6] qui est 
    % multipliée avec le vecteur des valeurs angulaires des articulations.
    % Ceci donnera le vecteur de rotaiton de l'assiette (et de ce fait du 
    % point de référence de la cabine). Ceci dans la convention NED.
    
    e6 = E1*E2*E3*E4*E5*[1 0 0]'; % axe x
    e5 = E1*E2*E3*E4*   [0 1 0]'; % axe y
    e4 = E1*E2*E3*      [1 0 0]'; % axe x
    e3 = E1*E2*         [0 1 0]'; % axe y
    e2 = E1*            [0 1 0]'; % axe y
    e1 = eye(3)*        [0 0 1]'; % axe z
    
    e = [e1 e2 e3 e4 e5 e6];
    
    % Afin de voir les changements sur Phi, Theta, Psi causés par les
    % vecteurs de rotations. Nous devons transformer le système "e" vers "b".
    % D'abord dans le tantage puis dans le alcet.
   
    % Quelques raccourcis pour accéler le temps de calcul
    cs_psi = cos(eul_ang(3));
    sn_psi = sin(eul_ang(3));
    cs_tet = cos(eul_ang(2));
    sn_tet = sin(eul_ang(2));
    
    PSI = [cs_psi sn_psi 0; -sn_psi cs_psi 0; 0 0 1];
    TET = [cs_tet 0 -sn_tet; 0 1 0; sn_tet 0 cs_tet];
    e = TET*PSI*e; % Redéfinition de "e" avec les changements sur Theta et Psi
    
    % Les dérivées de D1 à D6 pour chacune des articulations 
    dD1 = [-SA1 -CA1 0 0; CA1 -SA1 0 0; 0 0 0 0; 0 0 0 0];
    dD2 = [-SA2 0 CA2 0; 0 0 0 0; -CA2 0 -SA2 0; 0 0 0 0];
    dD3 = [-SA3 0 CA3 0; 0 0 0 0; -CA3 0 -SA3 0; 0 0 0 0];
    dD4 = [0 0 0 0; 0 -SA4 -CA4 0; 0 CA4 -SA4 0; 0 0 0 0];
    dD5 = [-SA5 0 CA5 0; 0 0 0 0; -CA5 0 -SA5 0; 0 0 0 0];
    dD6 = [0 0 0 0; 0 -SA6 -CA6 0; 0 CA6 -SA6 0; 0 0 0 0];
    
    % Nous créons la matrice "H": Hessien. L'inversion du Hessien détermine
    % la vitesse des articulations angualires telle une fonction des la
    % vitesse de (x,y,z) et de la vitesse des angles d'Euler.
    
    h1 = dD1*D2*D3*D4*D5*D6*x6;
    h2 = D1*dD2*D3*D4*D5*D6*x6;
    h3 = D1*D2*dD3*D4*D5*D6*x6;
    h4 = D1*D2*D3*dD4*D5*D6*x6;
    h5 = D1*D2*D3*D4*dD5*D6*x6;
    h6 = D1*D2*D3*D4*D5*dD6*x6;
    
    h = [h1 h2 h3 h4 h5 h6]; % Cette matrice [3x6] représente la moitié supérieure de "H"
    H = [h(1:3,:); e];       % La matrice [3x6] inférieure représnete la mtrice "e"
    
    d_ang = inv(H) * [( POS - pos );             % Valeur d'angles à ajouter 
                      (DTR*EUL_ANG - eul_ang)];  % aux valeurs initiales
          
    ang = ang + d_ang;       % Ajout de la valeur calculée à la valeur initiale                   
    
    ang = adjust_ang( ang ); % Appel de la fonction "adjust_ang" pour que
                             % l'angle soit compris dans [-pi,pi]
                             
    % Vérifications et calculs du nombre d'itération dans l'algorithme
    if(norm(d_ang) < 1.e-6)
        J_ANG = RTD*adjust_ang( ang );  % Appel de la fonction "adjust_ang" pour que
                                        % l'angle soit compris dans [-pi,pi]
                                        % Puis passage de [Rad] vers [°]
                                        
        Output(1,1)   = J_ANG(1);     % La sortie reçoit les nouvelles valeurs des 
        Output(2:5,1) = J_ANG(2:5);  % angles pour chacun des Thetas
        Output(6,1)   = J_ANG(6);     % Les - servent a base de NED a KUKA
        
        Output(7,1)   = N;      % La sortie reçoit également le nombre 
                                % d'itérations réalisées par l'algorithme
                                % pour converger vers une solution
        break;                  % En cas de réussite, on sort de la boucle
    end
    N = N + 1;    % si cette étape est réalisée, on incrémente le nombre
                  % d'itération de l'algorithme. 
    
    % Si nous effectuons plus de 10 itérations dans l'algorithme pour déterminer 
    % une solution, nous condisérons qu'il n'y a pas de convergence 
    if N > 100
        Output(1:6) = J_ANG_0; % return vector as is
        Output(7)   = -1;      % Code d'erreur: -1 <=> Pas de convergence
        return;
    end
end
%------------------------------
% FIN DE L'ALGORITHME ITERATIF 
%------------------------------
%% Mise en place de sécurité: les butées articulaires sont dépassées.
for i = 1 : 6
    if J_ANG(i) >= SL(1,i)
        Output(7,1) = -3;      % Code d'erreur: -3 <=> limite articulaire max dépassée
        min=i
        return;
    elseif J_ANG(i) <= SL(2,i)
        Output(7,1) = -3;      % Code d'erreur: -3 <=> limite articulaire min dépassée
        max=i
        return;
    end
end

end
